simulink model "suspn"  (Simulink 6.0)
settings: Solver=ode45  SolverMode=SingleTasking  StartTime=0.0  StopTime=10  MaxStep=0.01  RelTol=1e-3  AbsTol=1e-6
PreLoadFcn:
  | suspdat
values from neighbouring files (symbols this model uses):
  cf = 2500    [suspdat.m]
  cr = 2000    [suspdat.m]
  Iyy = 2100    [suspdat.m]
  kf = 28000    [suspdat.m]
  kr = 21000    [suspdat.m]
  Lf = 0.9    [suspdat.m]
  Lr = 1.2    [suspdat.m]
  Mb = 1200    [suspdat.m]
libraries: simulink x1
Description:
  | Cambridge Control, Ltd.
settings Model: Creator=The MathWorks Inc.  ModifiedByFormat=S. Quinn  LastModifiedBy=S. Quinn  ExtModeTrigMode=oneshot  ExtModeArmWhenConnect=off  ExtModeAutoUpdateStatusClock=off
settings DataIOCC: LimitDataPoints=off  SaveOutput=off  SaveState=on  StateSaveName=x  TimeSaveName=t
settings OptimizationCC: BooleanDataType=off
settings DebuggingCC: CheckExecutionContextPreStartOutputMsg=on  CheckExecutionContextRuntimeOutputMsg=on  SolverPrmCheckMsg=none  IntegerOverflowMsg=none
settings HardwareCC: TargetUnknown=on

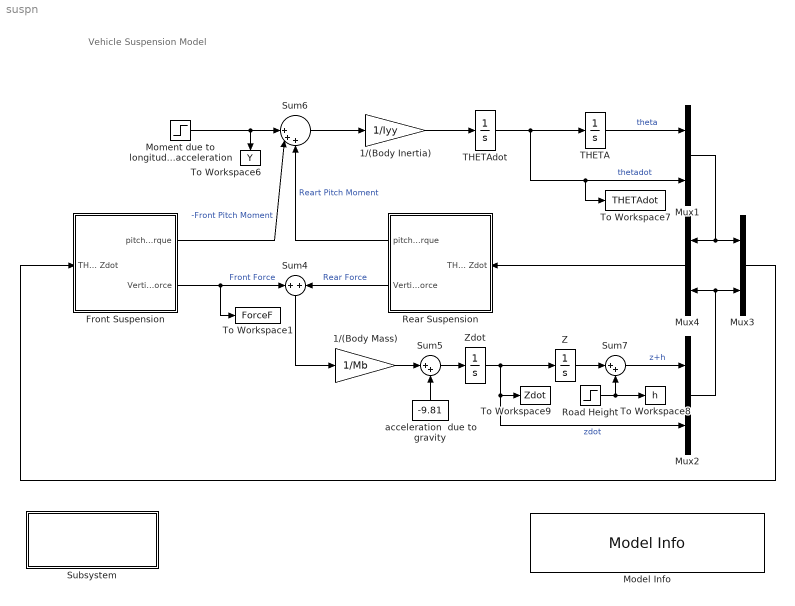
== system suspn ==
  note: Vehicle Suspension Model
  1/(Body Inertia) : Gain  Gain=1/Iyy  SaturateOnIntegerOverflow=on
  1/(Body Mass) : Gain  Gain=1/Mb  SaturateOnIntegerOverflow=on
  Front Suspension : Subsystem  PropExecContextAcrossSSBoundary=on  mask(half-car suspension){K=kf, C=cf, L=-Lf}
      mask prompts: K "Stiffness = spring rate:"; C "Damping rate:"; L "Moment arm:"
      mask help:
      | Half-Car Suspension
      | The spring and damping rates for an individual wheel are entered below.  Their combined effect as applied to two wheels at the specified distance from the center of mass is computed.  The distance should be specified as positive if the subsystem is oriented such that increasing z corresponds to increasing theta, negative otherwise.
      mask Help: See "Using Simulink and Stateflow in Automotive Applications" for a mathematical derivation of the subsystem operation.  Contact your MathWorks distributor to obtain a copy.
      mask Display: plot(-1, 0, 13, 12, [1 12], [11 11], [1 5], [2 2], [1 2], [4.5 5], [2 0], [5 6], [0 2], [6 7], [2 0], [7 8], [0 1], [8 8.5], [1 1], [8.5 11], [1 1], [2 4.5], [5 5], [2 5], [4 6], [5 5], [4 4], [5 8], [6 6], [5 8], [4 6], [6.5 6.5], [5 5], [6.5 11], [0 1], [1 2], [2 3], [1 2], [4 5], [1 2])
  Model Info : simulink/Model-Wide Utilities/Model Info  InitialBlockCM=none  BlockCM=none  Frame=on  DisplayStringWithTags=|  HorizontalTextAlignment=Center  LeftAlignmentValue=0.5  SourceBlockDiagram=suspn  TagMaxNumber=20
      | Two DOF Vehicle Suspension Model
      | %<Creator>
      | %<Description>
      | rev. %<ModifiedBy>  %<ModifiedDate>
  Moment due to longitudinal vehicle acceleration : Step  Time=3  After=100  SampleTime=0
  Mux1 : Mux  Inputs=2
      settings: DisplayOption=signals
  Mux2 : Mux  Inputs=2
      settings: DisplayOption=signals
  Mux3 : Mux  Inputs=2
      settings: DisplayOption=signals
  Mux4 : Mux  Orientation=left  Inputs=2
      settings: DisplayOption=signals
  Rear Suspension : Subsystem  Orientation=left  PropExecContextAcrossSSBoundary=on  mask(half-car suspension){K=kr, C=cr, L=Lr}
      mask prompts: K "Stiffness = spring rate:"; C "Damping rate:"; L "Moment arm:"
      mask help:
      | Half-Car Suspension
      | The spring and damping rates for an individual wheel are entered below.  Their combined effect as applied to two wheels at the specified distance from the center of mass is computed.  The distance should be specified as positive if the subsystem is oriented such that increasing z corresponds to increasing theta, negative otherwise.
      mask Help: See "Using Simulink and Stateflow in Automotive Applications" for a mathematical derivation of the subsystem operation.  Contact your MathWorks distributor to obtain a copy.
      mask Display: plot(-1, 0, 13, 12, [1 12], [11 11], [1 5], [2 2], [1 2], [4.5 5], [2 0], [5 6], [0 2], [6 7], [2 0], [7 8], [0 1], [8 8.5], [1 1], [8.5 11], [1 1], [2 4.5], [5 5], [2 5], [4 6], [5 5], [4 4], [5 8], [6 6], [5 8], [4 6], [6.5 6.5], [5 5], [6.5 11], [0 1], [1 2], [2 3], [1 2], [4 5], [1 2])
  Road Height : Step  Time=7  After=0.01  SampleTime=0
  Subsystem : Subsystem  PropExecContextAcrossSSBoundary=on
      settings: OpenFcn=suspgrph
      mask Display: disp('double-click to run\nthe simulation and\nplot the results')
  Sum4 : Sum  Orientation=down  SaturateOnIntegerOverflow=on  InputSameDT=on
  Sum5 : Sum  Inputs=|++  SaturateOnIntegerOverflow=on  InputSameDT=on
  Sum6 : Sum  Inputs=||+++  SaturateOnIntegerOverflow=on  InputSameDT=on
  Sum7 : Sum  Inputs=|++  SaturateOnIntegerOverflow=on  InputSameDT=on
  THETA : Integrator  InitialCondition=-8.7e-20
  THETAdot : Integrator  InitialCondition=8.04e-28
  To Workspace1 : ToWorkspace  VariableName=ForceF  SampleTime=0.01  SaveFormat=Array
      settings: MaxDataPoints=10e3
  To Workspace6 : ToWorkspace  VariableName=Y  SampleTime=0.01  SaveFormat=Array
      settings: Orientation=down  MaxDataPoints=10000
  To Workspace7 : ToWorkspace  VariableName=THETAdot  SampleTime=0.01  SaveFormat=Array
      settings: MaxDataPoints=10e3
  To Workspace8 : ToWorkspace  VariableName=h  SampleTime=0.01  SaveFormat=Array
      settings: MaxDataPoints=10e3
  To Workspace9 : ToWorkspace  VariableName=Zdot  SampleTime=0.01  SaveFormat=Array
      settings: MaxDataPoints=10e3
  Z : Integrator  InitialCondition=-0.12
  Zdot : Integrator
  acceleration  due to gravity : Constant  Orientation=up  Value=-9.81
  wires:
  Front Suspension/2(Vertical Force) -> Sum4/1, To Workspace1/1  "Front Force"
  Rear Suspension/2(Vertical Force) -> Sum4/2  "Rear Force"
  Sum4/1 -> 1/(Body Mass)/1
  Mux1/1 -> Mux3/1, Mux4/1
  Mux3/1 -> Front Suspension/1(THETA THETAdot Z Zdot)
  Mux4/1 -> Rear Suspension/1(THETA THETAdot Z Zdot)
  Sum5/1 -> Zdot/1
  acceleration  due to gravity/1 -> Sum5/2
  1/(Body Mass)/1 -> Sum5/1
  Z/1 -> Sum7/1
  Sum7/1 -> Mux2/1  "z+h"
  Zdot/1 -> Z/1, Mux2/2, To Workspace9/1  "zdot"
  Road Height/1 -> Sum7/2, To Workspace8/1
  Mux2/1 -> Mux3/2, Mux4/2
  Moment due to longitudinal vehicle acceleration/1 -> To Workspace6/1, Sum6/1
  Sum6/1 -> 1/(Body Inertia)/1
  Rear Suspension/1(pitch Torque) -> Sum6/3  "Reart Pitch Moment"
  Front Suspension/1(pitch Torque) -> Sum6/2  "-Front Pitch Moment"
  1/(Body Inertia)/1 -> THETAdot/1
  THETA/1 -> Mux1/1  "theta"
  THETAdot/1 -> THETA/1, To Workspace7/1, Mux1/2  "thetadot"

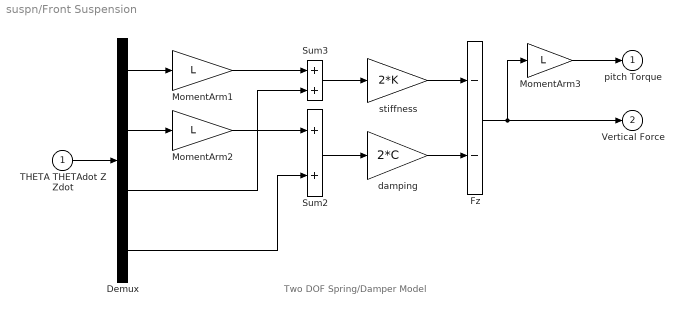
== system suspn/Front Suspension ==
  note: Two DOF Spring/Damper Model
  THETA THETAdot Z Zdot : Inport  Port=1  LatchInput=off
  Demux : Demux
  Fz : Sum  Inputs=--  SaturateOnIntegerOverflow=on  InputSameDT=on
  MomentArm1 : Gain  Gain=L  SaturateOnIntegerOverflow=on
  MomentArm2 : Gain  Gain=L  SaturateOnIntegerOverflow=on
  MomentArm3 : Gain  Gain=L  SaturateOnIntegerOverflow=on
  Sum2 : Sum  SaturateOnIntegerOverflow=on  InputSameDT=on
  Sum3 : Sum  SaturateOnIntegerOverflow=on  InputSameDT=on
  damping : Gain  Gain=2*C  SaturateOnIntegerOverflow=on
  stiffness : Gain  Gain=2*K  SaturateOnIntegerOverflow=on
  pitch Torque : Outport  InitialOutput=0
  Vertical Force : Outport  Port=2  InitialOutput=0
  wires:
  Sum2/1 -> damping/1
  Sum3/1 -> stiffness/1
  THETA THETAdot Z Zdot/1 -> Demux/1
  damping/1 -> Fz/2
  stiffness/1 -> Fz/1
  Fz/1 -> Vertical Force/1, MomentArm3/1
  MomentArm3/1 -> pitch Torque/1
  Demux/1 -> MomentArm1/1
  Demux/2 -> MomentArm2/1
  Demux/3 -> Sum3/2
  MomentArm1/1 -> Sum3/1
  MomentArm2/1 -> Sum2/1
  Demux/4 -> Sum2/2

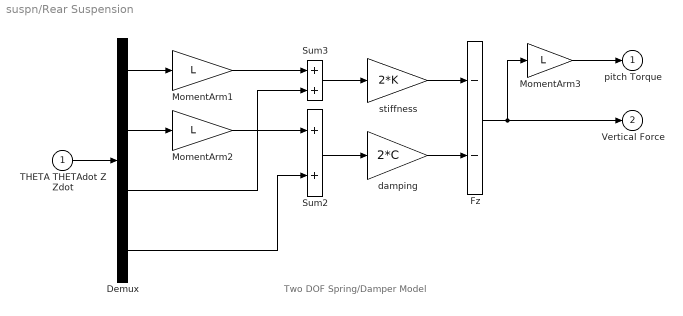
== system suspn/Rear Suspension ==
  note: Two DOF Spring/Damper Model
  THETA THETAdot Z Zdot : Inport  Port=1  LatchInput=off
  Demux : Demux
  Fz : Sum  Inputs=--  SaturateOnIntegerOverflow=on  InputSameDT=on
  MomentArm1 : Gain  Gain=L  SaturateOnIntegerOverflow=on
  MomentArm2 : Gain  Gain=L  SaturateOnIntegerOverflow=on
  MomentArm3 : Gain  Gain=L  SaturateOnIntegerOverflow=on
  Sum2 : Sum  SaturateOnIntegerOverflow=on  InputSameDT=on
  Sum3 : Sum  SaturateOnIntegerOverflow=on  InputSameDT=on
  damping : Gain  Gain=2*C  SaturateOnIntegerOverflow=on
  stiffness : Gain  Gain=2*K  SaturateOnIntegerOverflow=on
  pitch Torque : Outport  InitialOutput=0
  Vertical Force : Outport  Port=2  InitialOutput=0
  wires:
  Demux/4 -> Sum2/2
  MomentArm2/1 -> Sum2/1
  MomentArm1/1 -> Sum3/1
  Demux/3 -> Sum3/2
  Demux/2 -> MomentArm2/1
  Demux/1 -> MomentArm1/1
  MomentArm3/1 -> pitch Torque/1
  Fz/1 -> MomentArm3/1, Vertical Force/1
  stiffness/1 -> Fz/1
  damping/1 -> Fz/2
  THETA THETAdot Z Zdot/1 -> Demux/1
  Sum3/1 -> stiffness/1
  Sum2/1 -> damping/1

== system suspn/Subsystem ==
